simulink model "maquina_estados_test_slx"  (R2022b)
settings: Solver=VariableStepAuto  StartTime=0.0  StopTime=10e-4  RelTol=1e-3
libraries: hdlBasic x10, vmcUtilities x1
settings Model: Creator=adiglesias  LastModifiedBy=adiglesias

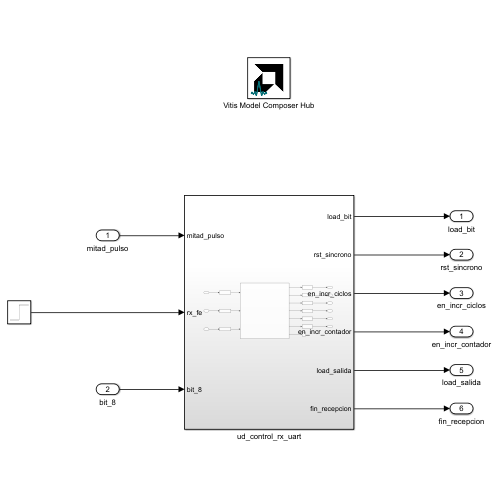
[thumbnail: Simulink's stored preview of the top-level diagram]
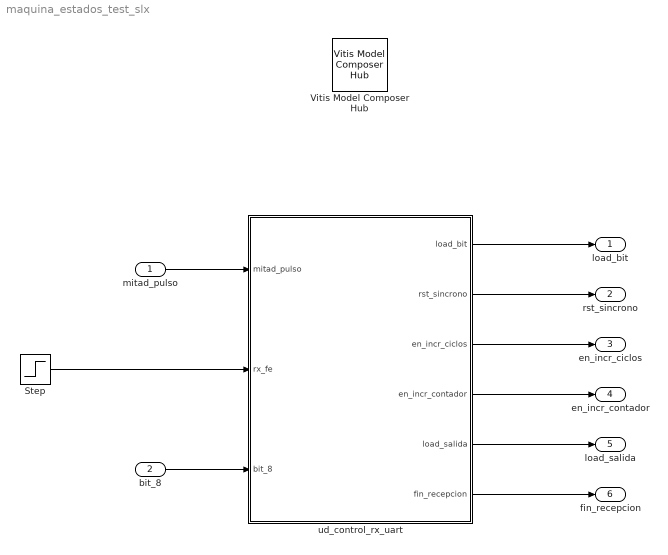
== system maquina_estados_test_slx ==
  mitad_pulso : Inport
  bit_8 : Inport  Port=2
  Step : Step  Time=1e-6  SampleTime=0
  Vitis Model Composer Hub : vmcUtilities/Vitis Model Composer Hub  Tag=genX  CodeGeneration=off  SubsystemName=ud_control_rx_uart  TargetDirectory=./code  ExportType=AI Engines  IpVendor=xilinx.com  IpLibrary=hls  IpVersion=1.0  IpHWLanguage=Verilog  AieCompilerOptions={}  AieSimulatorOptions={}  CreateTestbench=off  TestbenchStackSize=10  RunRtlSim=off  RunCSim=off  RunAieSim=off  AieSimTimeout=50000  RunAieSimProfiling=off  LaunchVitisAnalyzer=off  PlotOutput=off  RunX86Sim=off  X86SimTimeout=10  GenHwImage=off  GenLibadfXo=off  PlatformType=Not Specified  HwSystemType=Baremetal  HwValidationTarget=hw  ProjDevice=Zynq UltraScale+ RFSoC ZCU208 Evaluation Kit (xczu48dr-fsvg1517-2-e)  ProjDevicePart=xczu48dr-fsvg1517-2-e  AIEType=None  SamplePeriod=-1  ClockFrequency=200  DataPathParallelism=1  xilinxfamily=zynquplusRFSOC  part=xczu48dr  speed=-2-e  package=fsvg1517  directory=./code\ip\ud_control_rx_uart\src  testbench=off  incr_netlist=off  synthesis_tool=Vivado  clock_wrapper=Clock Enables  dbl_ovrd=According to Block Masks  dcm_input_clock_period=10  sysclk_period=10  simulink_period=1/100e6  eval_field=0  LogFileName=''  NThreads=4
  ud_control_rx_uart : Subsystem
  load_bit : Outport
  rst_sincrono : Outport  Port=2
  en_incr_ciclos : Outport  Port=3
  en_incr_contador : Outport  Port=4
  load_salida : Outport  Port=5
  fin_recepcion : Outport  Port=6
  wires:
  bit_8/1 -> ud_control_rx_uart/3(bit_8)
  Step/1 -> ud_control_rx_uart/2(rx_fe)
  mitad_pulso/1 -> ud_control_rx_uart/1(mitad_pulso)
  ud_control_rx_uart/5(load_salida) -> load_salida/1
  ud_control_rx_uart/3(en_incr_ciclos) -> en_incr_ciclos/1
  ud_control_rx_uart/1(load_bit) -> load_bit/1
  ud_control_rx_uart/4(en_incr_contador) -> en_incr_contador/1
  ud_control_rx_uart/2(rst_sincrono) -> rst_sincrono/1
  ud_control_rx_uart/6(fin_recepcion) -> fin_recepcion/1

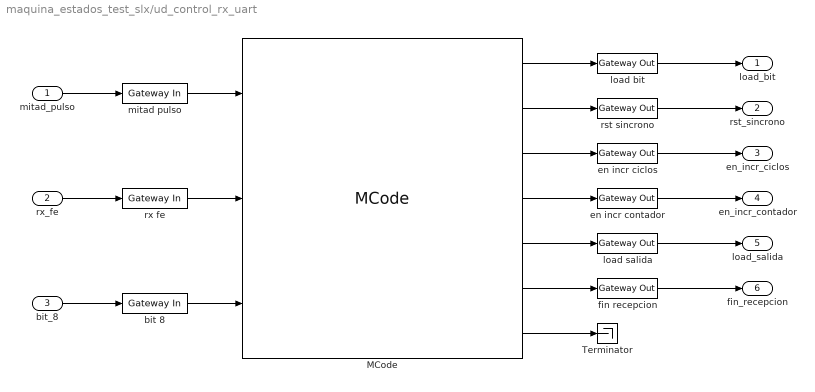
== system maquina_estados_test_slx/ud_control_rx_uart ==
  mitad_pulso : Inport
  rx_fe : Inport  Port=2
  bit_8 : Inport  Port=3
  MCode : hdlBasic/MCode  mfname=state_machine  explicit_period=off  period=1  iptable={ 'mitad_pulso', ''; 'rx_fe', ''; 'bit_8', '' }  optable={ 'load_bit', 'off'; 'rst_sincrono', 'off'; 'en_incr_ciclos', 'off'; 'en_incr_contador', 'off'; 'load_salida', 'off'; 'fin_recepcion', 'off'; 'estado_actual', 'off' }  enable_stdout=off  enable_debug=off  suppress_output='on'  defparams={}  hide_port_list={}  block_type=mcode  block_width=444  block_height=788
      settings: infoedit=Pass input values to a MATLAB function for evaluation in Xilinx fixed-point type. The input ports of the block are input arguments of the function. The output ports of the block are output arguments of the function.
  Terminator : Terminator
  bit 8 : hdlBasic/Gateway In  gui_display_data_type=Fixed-point  arith_type=Unsigned  n_bits=1  bin_pt=0  preci_type=Single  exp_width=8  frac_width=24  rows=1  columns=1  quantization="Round  (unbiased: +/- Inf)"  overflow=Saturate  period=10e-9  UseAsADC=off  ADCChannel='1'  interface=None  automatic_assignment=on  address_offset=hex2dec('00')  intf_name=''  intf_description=''  default_value=0  timing_constraint=None  locs_specified=off  LOCs={}  io_standard={}  inherit_from_input=off  hdl_port=on  XmcBlockStatus=1  maskContainerNames=group4  block_type=gatewayin  block_config=sysgen:gateway_in_config  block_width_w=590  block_height_w=620  block_width=640  block_height=850
  en incr ciclos : hdlBasic/Gateway Out  inherit_from_input=off  hdl_port=on  rows=1  columns=1  UseAsDAC=off  DACChannel='1'  interface=None  automatic_assignment=on  address_offset=hex2dec('00')  intf_name=''  intf_description=''  timing_constraint=None  locs_specified=off  LOCs={}  io_standard={}  XmcBlockStatus=1  maskContainerNames=group4  block_type=gatewayout  block_config=sysgen:gateway_out_config  block_width_w=590  block_height_w=620  block_width=620  block_height=750
  en incr contador : hdlBasic/Gateway Out  inherit_from_input=off  hdl_port=on  rows=1  columns=1  UseAsDAC=off  DACChannel='1'  interface=None  automatic_assignment=on  address_offset=hex2dec('00')  intf_name=''  intf_description=''  timing_constraint=None  locs_specified=off  LOCs={}  io_standard={}  XmcBlockStatus=1  maskContainerNames=group4  block_type=gatewayout  block_config=sysgen:gateway_out_config  block_width_w=590  block_height_w=620  block_width=620  block_height=750
  fin recepcion : hdlBasic/Gateway Out  inherit_from_input=off  hdl_port=on  rows=1  columns=1  UseAsDAC=off  DACChannel='1'  interface=None  automatic_assignment=on  address_offset=hex2dec('00')  intf_name=''  intf_description=''  timing_constraint=None  locs_specified=off  LOCs={}  io_standard={}  XmcBlockStatus=1  maskContainerNames=group4  block_type=gatewayout  block_config=sysgen:gateway_out_config  block_width_w=590  block_height_w=620  block_width=620  block_height=750
  load bit : hdlBasic/Gateway Out  inherit_from_input=off  hdl_port=on  rows=1  columns=1  UseAsDAC=off  DACChannel='1'  interface=None  automatic_assignment=on  address_offset=hex2dec('00')  intf_name=''  intf_description=''  timing_constraint=None  locs_specified=off  LOCs={}  io_standard={}  XmcBlockStatus=1  maskContainerNames=group4  block_type=gatewayout  block_config=sysgen:gateway_out_config  block_width_w=590  block_height_w=620  block_width=620  block_height=750
  load salida : hdlBasic/Gateway Out  inherit_from_input=off  hdl_port=on  rows=1  columns=1  UseAsDAC=off  DACChannel='1'  interface=None  automatic_assignment=on  address_offset=hex2dec('00')  intf_name=''  intf_description=''  timing_constraint=None  locs_specified=off  LOCs={}  io_standard={}  XmcBlockStatus=1  maskContainerNames=group4  block_type=gatewayout  block_config=sysgen:gateway_out_config  block_width_w=590  block_height_w=620  block_width=620  block_height=750
  mitad pulso : hdlBasic/Gateway In  gui_display_data_type=Fixed-point  arith_type=Unsigned  n_bits=1  bin_pt=0  preci_type=Single  exp_width=8  frac_width=24  rows=1  columns=1  quantization="Round  (unbiased: +/- Inf)"  overflow=Saturate  period=10e-9  UseAsADC=off  ADCChannel='1'  interface=None  automatic_assignment=on  address_offset=hex2dec('00')  intf_name=''  intf_description=''  default_value=0  timing_constraint=None  locs_specified=off  LOCs={}  io_standard={}  inherit_from_input=off  hdl_port=on  XmcBlockStatus=1  maskContainerNames=group4  block_type=gatewayin  block_config=sysgen:gateway_in_config  block_width_w=590  block_height_w=620  block_width=640  block_height=850
  rst sincrono : hdlBasic/Gateway Out  inherit_from_input=off  hdl_port=on  rows=1  columns=1  UseAsDAC=off  DACChannel='1'  interface=None  automatic_assignment=on  address_offset=hex2dec('00')  intf_name=''  intf_description=''  timing_constraint=None  locs_specified=off  LOCs={}  io_standard={}  XmcBlockStatus=1  maskContainerNames=group4  block_type=gatewayout  block_config=sysgen:gateway_out_config  block_width_w=590  block_height_w=620  block_width=620  block_height=750
  rx fe : hdlBasic/Gateway In  gui_display_data_type=Fixed-point  arith_type=Unsigned  n_bits=1  bin_pt=0  preci_type=Single  exp_width=8  frac_width=24  rows=1  columns=1  quantization="Round  (unbiased: +/- Inf)"  overflow=Saturate  period=10e-9  UseAsADC=off  ADCChannel='1'  interface=None  automatic_assignment=on  address_offset=hex2dec('00')  intf_name=''  intf_description=''  default_value=0  timing_constraint=None  locs_specified=off  LOCs={}  io_standard={}  inherit_from_input=off  hdl_port=on  XmcBlockStatus=1  maskContainerNames=group4  block_type=gatewayin  block_config=sysgen:gateway_in_config  block_width_w=590  block_height_w=620  block_width=640  block_height=850
  load_bit : Outport
  rst_sincrono : Outport  Port=2
  en_incr_ciclos : Outport  Port=3
  en_incr_contador : Outport  Port=4
  load_salida : Outport  Port=5
  fin_recepcion : Outport  Port=6
  wires:
  MCode/2 -> rst sincrono/1
  load bit/1 -> load_bit/1
  rst sincrono/1 -> rst_sincrono/1
  mitad_pulso/1 -> mitad pulso/1
  load salida/1 -> load_salida/1
  en incr ciclos/1 -> en_incr_ciclos/1
  bit_8/1 -> bit 8/1
  MCode/4 -> en incr contador/1
  bit 8/1 -> MCode/3
  fin recepcion/1 -> fin_recepcion/1
  MCode/1 -> load bit/1
  MCode/5 -> load salida/1
  mitad pulso/1 -> MCode/1
  MCode/7 -> Terminator/1
  MCode/6 -> fin recepcion/1
  rx_fe/1 -> rx fe/1
  en incr contador/1 -> en_incr_contador/1
  rx fe/1 -> MCode/2
  MCode/3 -> en incr ciclos/1
